simulink model "blocks"  (R2019a)
settings: Solver=VariableStepAuto  StartTime=0.0  StopTime=10.0  RelTol=1e-3
settings Model: Creator=adeye  LastModifiedBy=adeye

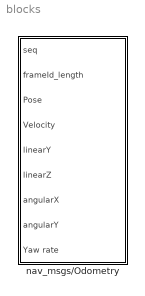
== system blocks ==
  nav_msgs/Odometry : Subsystem  mask{topic='/vehicle/odom', message_type='nav_msgs/Odometry', port=9090, timeout=2}
      mask prompts: topic "Topic name"; message_type "Message type"; timeout "Timeout (s)"

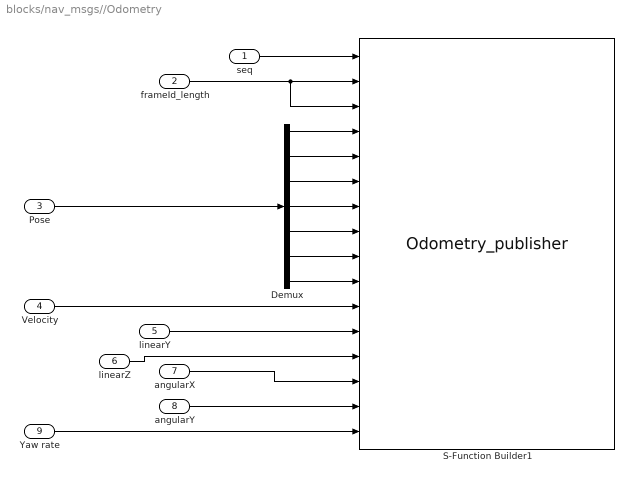
== system blocks/nav_msgs//Odometry ==
  seq : Inport
  frameId_length : Inport  Port=2
  Pose : Inport  Port=3
  Velocity : Inport  Port=4
  linearY : Inport  Port=5
  linearZ : Inport  Port=6
  angularX : Inport  Port=7
  angularY : Inport  Port=8
  Yaw rate : Inport  Port=9
  Demux : Demux  Outputs=7
  S-Function Builder1 : S-Function  InitFcn=try, set_param(gcb,'FunctionName','Odometry_publisher'), end  FunctionName=Odometry_publisher  Parameters=int8(topic),int8(message_type),port,timeout  SFunctionModules=Odometry_publisher_wrapper rosbridge_functions  SFunctionDeploymentMode=off  EnableBusSupport=off  mask(S-Function Builder){}
      mask help: Simulink:masks:SFunctionBuilder_MD
      mask init:
      | val = [[.9  0.75 0.75 1 1 .9 .9 1]',[1 1 0.75 0.75 .9 .9 1 .9]'];try , sys = get_param(gcb,'SfunBuilderFcnName');if isempty(sys), sys = get_param(gcb,'FunctionName'); end,catch, sys = get_param(gcb,'FunctionName'); end
      settings: CopyFcn=set_param(gcbh,'LinkStatus','none')  PreSaveFcn=try, set_param(gcb,'FunctionName','Odometry_publisher'), end  OpenFcn=sfunctionwizard(gcbh)
      mask Display: plot(val(:,1),val(:,2)),disp(sys), port_label('input',1,'seq'), port_label('input',2,'frameId_length'), port_label('input',3,'childFrameId_length'), port_label('input',4,'positionX'), port_label('input',5,'positionY'), port_label('input',6,'positionZ'), port_label('input',7,'orientW'), port_label('input',8,'orientX'), port_label('input',9,'orientY'), port_label('input',10,'orientZ'), port_label('input',11,'linearX'), port_label('input',12,'linearY'), port_label('input',13,'linearZ'), port_label('input',14,'angularX'), port_label('input',15,'angularY'), port_label('input',16,'angularZ')
  wires:
  Demux/5 -> S-Function Builder1/8
  Pose/1 -> Demux/1
  Demux/4 -> S-Function Builder1/7
  Demux/7 -> S-Function Builder1/10
  Demux/1 -> S-Function Builder1/4
  Demux/2 -> S-Function Builder1/5
  Demux/3 -> S-Function Builder1/6
  Demux/6 -> S-Function Builder1/9
  Velocity/1 -> S-Function Builder1/11
  Yaw rate/1 -> S-Function Builder1/16
  seq/1 -> S-Function Builder1/1
  frameId_length/1 -> S-Function Builder1/3, S-Function Builder1/2
  linearY/1 -> S-Function Builder1/12
  linearZ/1 -> S-Function Builder1/13
  angularX/1 -> S-Function Builder1/14
  angularY/1 -> S-Function Builder1/15
